simulink model "lesson_1"  (R2016a)
settings: Solver=VariableStepAuto  StartTime=0.0  StopTime=10.0  RelTol=1e-3
values from neighbouring files (symbols this model uses):
  D = 1e-3    (= 0.001)    [initialization_for_lesson1.m]    (also in initialization_for_lesson4.m; initialization_for_lesson5.m)
  f = 50    [initialization_for_lesson1.m]    (also in initialization_for_lesson2.m; initialization_for_lesson4.m; initialization_for_lesson5.m)
  Fs = Vs*sqrt(2/3)/(2*pi*f)    [initialization_for_lesson1.m]    (also in initialization_for_lesson2.m = ims*Lm; initialization_for_lesson4.m; initialization_for_lesson5.m)
  fsw = 4e3    (= 4000)    [initialization_for_lesson1.m]    (also in initialization_for_lesson4.m; initialization_for_lesson5.m)
  J = 127    [initialization_for_lesson1.m]    (also in initialization_for_lesson4.m; initialization_for_lesson5.m)
  ki_id = (wni^2)*Lr*sigma    (= 491.599501999)    [initialization_for_lesson1.m]    (also in initialization_for_lesson4.m; initialization_for_lesson5.m)
  ki_iq = ki_id    (= 491.599501999)    [initialization_for_lesson1.m]    (also in initialization_for_lesson4.m; initialization_for_lesson5.m)
  ki_n = ((wnn^2)*J)/p    (= 25400)    [initialization_for_lesson1.m]    (also in initialization_for_lesson4.m = 406400; initialization_for_lesson5.m = 406400)
  kp_id = (2*wni*sigma*Lr)-Rr    (= 0.5771)    [initialization_for_lesson1.m]    (also in initialization_for_lesson4.m; initialization_for_lesson5.m)
  kp_iq = kp_id    (= 0.5771)    [initialization_for_lesson1.m]    (also in initialization_for_lesson4.m; initialization_for_lesson5.m)
  kp_n = (2*wnn*J)/p    (= 2540)    [initialization_for_lesson1.m]    (also in initialization_for_lesson4.m = 10160; initialization_for_lesson5.m = 10160)
  Lm = 2.5e-3    (= 0.0025)    [initialization_for_lesson1.m]    (also in initialization_for_lesson2.m; initialization_for_lesson4.m; initialization_for_lesson5.m)
  Lr = Lm + Lsi    (= 0.002587)    [initialization_for_lesson1.m]    (also in initialization_for_lesson2.m; initialization_for_lesson4.m; initialization_for_lesson5.m)
  Ls = Lm + Lsi    (= 0.002587)    [initialization_for_lesson1.m]    (also in initialization_for_lesson2.m; initialization_for_lesson4.m; initialization_for_lesson5.m)
  Lsi = 0.087e-3    (= 8.7e-05)    [initialization_for_lesson1.m]    (also in initialization_for_lesson2.m; initialization_for_lesson4.m; initialization_for_lesson5.m)
  p = 2    [initialization_for_lesson1.m]    (also in initialization_for_lesson2.m; initialization_for_lesson4.m; initialization_for_lesson5.m)
  Ps = 2e6    (= 2000000)    [initialization_for_lesson1.m]    (also in initialization_for_lesson2.m; initialization_for_lesson4.m; initialization_for_lesson5.m)
  Rr = 2.9e-3    (= 0.0029)    [initialization_for_lesson1.m]    (also in initialization_for_lesson2.m; initialization_for_lesson4.m; initialization_for_lesson5.m)
  Rs = 2.6e-3    (= 0.0026)    [initialization_for_lesson1.m]    (also in initialization_for_lesson2.m; initialization_for_lesson4.m; initialization_for_lesson5.m)
  sigma = 1 - Lm^2/(Ls*Lr)    (= 0.0661284179513)    [initialization_for_lesson1.m]    (also in initialization_for_lesson2.m; initialization_for_lesson4.m; initialization_for_lesson5.m)
  Tem = 12732    [initialization_for_lesson1.m]    (also in initialization_for_lesson2.m = Temm(i); initialization_for_lesson4.m; initialization_for_lesson5.m)
  Ts = 1/fsw/50    (= 5e-06)    [initialization_for_lesson1.m]    (also in initialization_for_lesson4.m; initialization_for_lesson5.m)
  Vbus = Vr_stator*sqrt(2)    [initialization_for_lesson1.m]    (also in initialization_for_lesson2.m; initialization_for_lesson4.m; initialization_for_lesson5.m)
  Vs = 690    [initialization_for_lesson1.m]    (also in initialization_for_lesson2.m = 690*sqrt(2/3); initialization_for_lesson4.m; initialization_for_lesson5.m)
undefined symbols (not defined in the file or in its folder): DiscIntNeverNeededParam
libraries: powerlib x8, powerlib_meascontrol x1
settings Model: Creator=EBUKA  LastModifiedBy=EBUKA
settings GRTTargetCC: GeneratePreprocessorConditionals=Use local settings

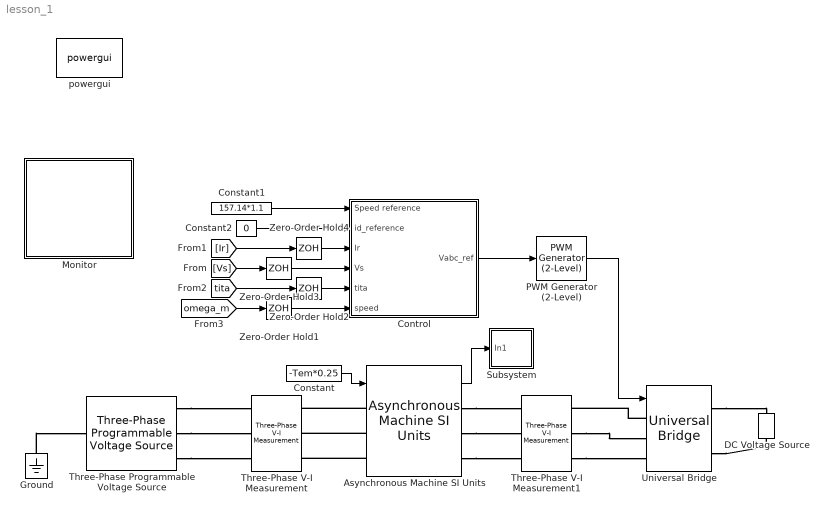
== system lesson_1 ==
  Asynchronous Machine SI Units : powerlib/Machines/Asynchronous Machine SI Units  RotorType=Wound  PresetModel=No  MechanicalLoad=Torque Tm  ShowDetailedParameters=on  ReferenceFrame=Rotor  Units=SI  MeasurementBus=off  NominalParameters=[Ps Vs f]  Stator=[Rs, Lsi]  Rotor=[Rr, Lsi]  Cage1=[0.4155 0.002066]  Cage2=[0.4168 0.0003495]  Lm=Lm  Mechanical=[J D 2]  PolePairs=2  InitialConditions=[1 0 0 0 0 0 0 0]  SimulateSaturation=off  Saturation=[14.03593122, 27.81365428, 53.79336849, 72.68890987, 97.98006896, 148.6815601, 215.7428561, 302.9841135, 428.7778367 ; 230, 322, 414, 460, 506, 552, 598, 644, 690]  LoadFlowParameters=1492000  TsPowergui=0  TsBlock=-1  IterativeModel=Trapezoidal non iterative  IterativeDiscreteModel=Trapezoidal non iterative  Pmec=1.492e+006
  Constant : Constant  Value=-Tem*0.25
  Constant1 : Constant  Value=157.14*1.1
  Constant2 : Constant  Value=0
  Control : Subsystem
  DC Voltage Source : powerlib/Electrical Sources/DC Voltage Source  Amplitude=Vbus  Measurements=None
  Ground : powerlib/Elements/Ground  LConnTagsString=a
  Monitor : Subsystem
  PWM Generator (2-Level) : powerlib_meascontrol/Pulse & Signal Generators/PWM Generator (2-Level)  ModulatorType=Three-phase bridge (6 pulses)  ModulatorMode=Unsynchronized  Fc=fsw  Pc=90  nF=27  MinMax="[ -1  1 ]"  SamplingTechnique=Symmetrical regular (single edge)  ModulatingSignals=off  m=0.8  Freq=60  Phase=0  Ts=0  ShowCarrierOutport=off
  Subsystem : Subsystem
  Three-Phase Programmable Voltage Source : powerlib/Electrical Sources/Three-Phase Programmable Voltage Source  PositiveSequence="[Vs  0 f]"  VariationEntity=None  VariationType=Table of time-amplitude pairs  VariationTypeAlt=Step  VariationStep=0.5  VariationRate=10  VariationMagnitude=0.3  VariationFrequency=2  VariationTiming=[1 2]  VariationPhaseA=off  Amplitudes=[1 0.8 1.2 1.0]  TimeValues=[0 0.1 0.15 0.2]  HarmonicGeneration=off  HarmonicA=[3 0.2 -25 0]  HarmonicB=[2 0.15 35 2]  Timing="[0.05  3]"  BusType=swing  Pref=0  Qref=0  Qmin=-inf  Qmax=inf
  Three-Phase V-I Measurement : powerlib/Measurements/Three-Phase V-I Measurement  VoltageMeasurement=phase-to-ground  SetLabelV=on  LabelV=Vs  Vpu=on  VpuLL=off  CurrentMeasurement=yes  SetLabelI=on  LabelI=Is  Ipu=off  Pbase=100e6  Vbase=500e3  OutputType=Complex  PhasorSimulation=off  PSBequivalent=0
  Three-Phase V-I Measurement1 : powerlib/Measurements/Three-Phase V-I Measurement  VoltageMeasurement=no  SetLabelV=off  LabelV=Vs  Vpu=off  VpuLL=off  CurrentMeasurement=yes  SetLabelI=on  LabelI=Ir  Ipu=off  Pbase=100e6  Vbase=500e3  OutputType=Complex  PhasorSimulation=off  PSBequivalent=0
  Universal Bridge : powerlib/Power Electronics/Universal Bridge  Arms=3  SnubberResistance=1e5  SnubberCapacitance=inf  Device=Ideal Switches  Ron=1e-3  Lon=0  ForwardVoltages="[  0  0  ]"  ForwardVoltage=0  GTOparameters=[ 10e-6 , 20e-6 ]  IGBTparameters=[ 1e-6 , 2e-6 ]  Measurements=None  Measurements_2=None  converterType=Rectifier
  Zero-Order Hold{1..4} (4 alike) : ZeroOrderHold  SampleTime=1/fsw
  powergui : powerlib/powergui  Priority=1  SimulationMode=Discrete  SolverType=Tustin/Backward Euler (TBE)  SampleTime=Ts  frequency=60  SPID=off  DisableSnubberDevices=off  DisableRonSwitches=off  DisableVfSwitches=off  SwTol=0  DisplayEquations=off  Interpol=off  ExternalGateDelay=off  methode=off  Ts=10  FunctionMessages=off  echomessages=off  HookPort=off  EnableUseOfTLC=off  x0status=blocks  frequencyindice=50  Pbase=100e6  ErrMax=1e-4  Iterations=50  UnitsV=kV  UnitsW=MW  buscounter=0  RestoreLinks=warning  ResistiveCurrentMeasurement=off  Frange=[0:2:500]  Ylog=off  Xlog=on  ShowGrid=off  save=off  variable=ZData  structure=0  ZoomFFT=off  StartTime=0.0  cycles=1  DisplayStyle=1  fundamental=60  FreqAxis=off  MaxFrequency=1000  frequencyindicesteady=1  RmsSteady=1  display=off
  wires:
  Constant/1 -> Asynchronous Machine SI Units/1
  PWM Generator (2-Level)/1 -> Universal Bridge/1
  Control/1(Vabc_ref) -> PWM Generator (2-Level)/1
  Constant1/1 -> Control/1(Speed reference)
  Constant2/1 -> Control/2(id_reference)
  [Vs] -> Zero-Order Hold3/1
  [Ir] -> Zero-Order Hold4/1
  Asynchronous Machine SI Units/1 -> Subsystem/1(In1)
  [tita] -> Zero-Order Hold2/1
  [omega_m] -> Zero-Order Hold1/1
  Zero-Order Hold2/1 -> Control/5(tita)
  Zero-Order Hold1/1 -> Control/6(speed)
  Zero-Order Hold3/1 -> Control/4(Vs)
  Zero-Order Hold4/1 -> Control/3(Ir)
  connections:
  Asynchronous Machine SI Units/LConn1 -- Three-Phase V-I Measurement/RConn1
  Asynchronous Machine SI Units/LConn2 -- Three-Phase V-I Measurement/RConn2
  Asynchronous Machine SI Units/LConn3 -- Three-Phase V-I Measurement/RConn3
  Three-Phase Programmable Voltage Source/RConn1 -- Three-Phase V-I Measurement/LConn1
  Three-Phase Programmable Voltage Source/RConn2 -- Three-Phase V-I Measurement/LConn2
  Three-Phase Programmable Voltage Source/RConn3 -- Three-Phase V-I Measurement/LConn3
  Ground/LConn1 -- Three-Phase Programmable Voltage Source/LConn1
  Universal Bridge/RConn2 -- DC Voltage Source/LConn1
  Universal Bridge/RConn1 -- DC Voltage Source/RConn1
  Asynchronous Machine SI Units/RConn1 -- Three-Phase V-I Measurement1/RConn1
  Asynchronous Machine SI Units/RConn2 -- Three-Phase V-I Measurement1/RConn2
  Asynchronous Machine SI Units/RConn3 -- Three-Phase V-I Measurement1/RConn3
  Universal Bridge/LConn1 -- Three-Phase V-I Measurement1/LConn1
  Three-Phase V-I Measurement1/LConn2 -- Universal Bridge/LConn2
  Three-Phase V-I Measurement1/LConn3 -- Universal Bridge/LConn3

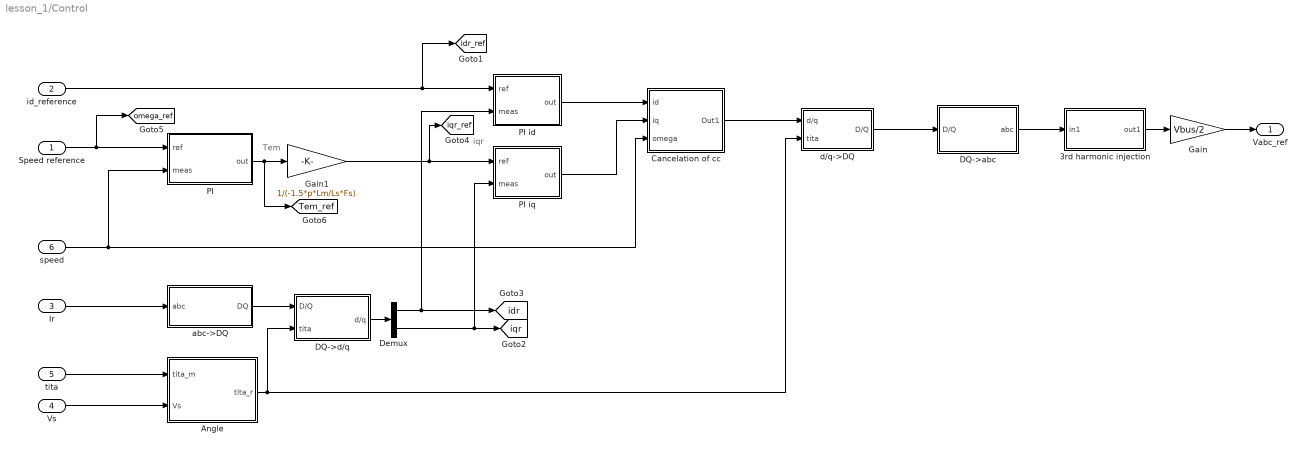
== system lesson_1/Control ==
  note: iqr
  note: Tem
  Speed reference : Inport
  id_reference : Inport  Port=2
  Ir : Inport  Port=3
  Vs : Inport  Port=4
  tita : Inport  Port=5
  speed : Inport  Port=6
  3rd harmonic injection : Subsystem
  Angle : Subsystem
  Cancelation of cc : Subsystem
  DQ->abc : Subsystem
  DQ->d/q : Subsystem
  Demux : Demux  Outputs=2
  Gain : Gain  Gain=Vbus/2
  Gain1 : Gain  Gain=1/(-1.5*p*Lm/Ls*Fs)
  PI : Subsystem
  PI id : Subsystem
  PI iq : Subsystem
  abc->DQ : Subsystem
  d/q->DQ : Subsystem
  Vabc_ref : Outport
  tag scope: Tem_ref=global, idr=global, idr_ref=global, iqr=global, iqr_ref=global, omega_ref=global
  wires:
  DQ->abc/1(abc) -> 3rd harmonic injection/1(in1)
  Gain/1 -> Vabc_ref/1
  d/q->DQ/1(D/Q) -> DQ->abc/1(D/Q)
  Ir/1 -> abc->DQ/1(abc)
  abc->DQ/1(DQ) -> DQ->d/q/1(D/Q)
  3rd harmonic injection/1(out1) -> Gain/1
  tita/1 -> Angle/1(tita_m)
  Vs/1 -> Angle/2(Vs)
  PI id/1(out) -> Cancelation of cc/1(id)
  PI iq/1(out) -> Cancelation of cc/2(iq)
  speed/1 -> PI/2(meas), Cancelation of cc/3(omega)
  Cancelation of cc/1(Out1) -> d/q->DQ/1(d/q)
  DQ->d/q/1(d/q) -> Demux/1
  Demux/1 -> [idr], PI id/2(meas)
  Demux/2 -> [iqr], PI iq/2(meas)
  Speed reference/1 -> [omega_ref], PI/1(ref)
  Angle/1(tita_r) -> d/q->DQ/2(tita), DQ->d/q/2(tita)
  PI/1(out) -> [Tem_ref], Gain1/1
  Gain1/1 -> [iqr_ref], PI iq/1(ref)
  id_reference/1 -> [idr_ref], PI id/1(ref)

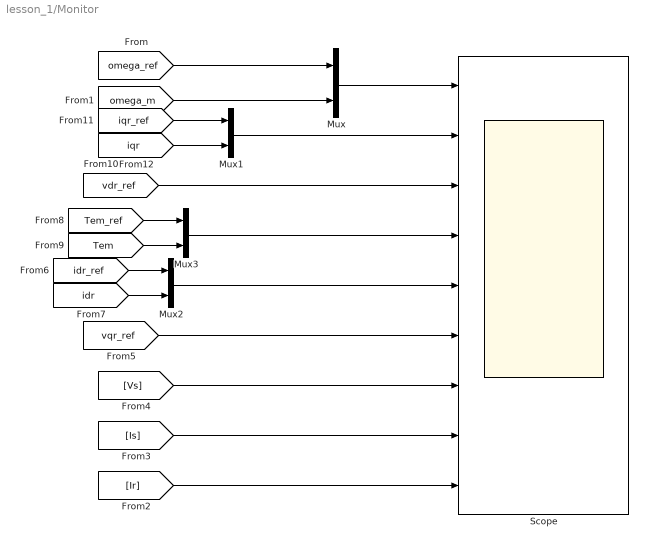
== system lesson_1/Monitor ==
  Mux{,1..3} (4 alike) : Mux  Inputs=2
  Scope : Scope  NumInputPorts=9
  wires:
  [omega_ref] -> Mux/1
  [omega_m] -> Mux/2
  [Ir] -> Scope/9
  [Is] -> Scope/8
  [Vs] -> Scope/7
  [idr_ref] -> Mux2/1
  [idr] -> Mux2/2
  Mux3/1 -> Scope/4
  [Tem_ref] -> Mux3/1
  [Tem] -> Mux3/2
  [vdr_ref] -> Scope/3
  [iqr_ref] -> Mux1/1
  [iqr] -> Mux1/2
  Mux1/1 -> Scope/2
  Mux2/1 -> Scope/5
  [vqr_ref] -> Scope/6
  Mux/1 -> Scope/1

== system lesson_1/Subsystem ==
  In1 : Inport
  Bus Selector : BusSelector  OutputSignals=Mechanical.Rotor angle thetam (rad),Mechanical.Rotor speed (wm),Mechanical.Electromagnetic torque Te (N*m)
  tag scope: Tem=global, omega_m=global, tita=global
  wires:
  In1/1 -> Bus Selector/1
  Bus Selector/2 -> [omega_m]  "<Rotor speed (wm)>"
  Bus Selector/1 -> [tita]  "<Rotor angle thetam (rad)>"
  Bus Selector/3 -> [Tem]  "<Electromagnetic torque Te (N*m)>"

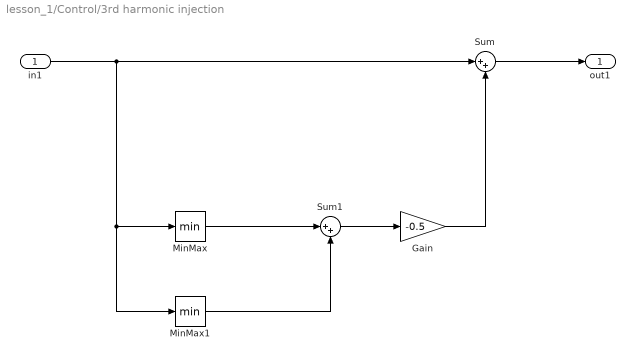
== system lesson_1/Control/3rd harmonic injection ==
  in1 : Inport
  Gain : Gain  Gain=-0.5
  MinMax : MinMax
  MinMax1 : MinMax
  Sum : Sum  Inputs=|++
  Sum1 : Sum  Inputs=|++
  out1 : Outport
  wires:
  Sum/1 -> out1/1
  in1/1 -> MinMax1/1, MinMax/1, Sum/1
  Gain/1 -> Sum/2
  Sum1/1 -> Gain/1
  MinMax/1 -> Sum1/1
  MinMax1/1 -> Sum1/2

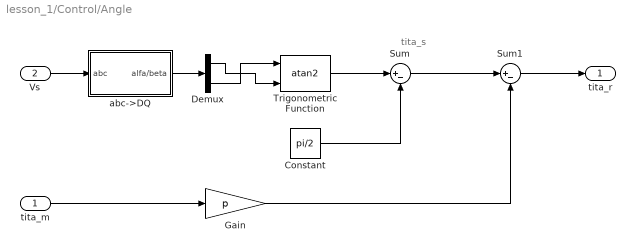
== system lesson_1/Control/Angle ==
  note: tita_s
  tita_m : Inport
  Vs : Inport  Port=2
  Constant : Constant  Value=pi/2
  Demux : Demux  Outputs=2
  Gain : Gain  Gain=p
  Sum : Sum  Inputs=|+-
  Sum1 : Sum  Inputs=|+-
  Trigonometric Function : Trigonometry  Operator=atan2
  abc->DQ : Subsystem
  tita_r : Outport
  wires:
  Vs/1 -> abc->DQ/1(abc)
  abc->DQ/1(alfa/beta) -> Demux/1
  Demux/2 -> Trigonometric Function/1
  Demux/1 -> Trigonometric Function/2
  Trigonometric Function/1 -> Sum/1
  Constant/1 -> Sum/2
  Sum/1 -> Sum1/1
  tita_m/1 -> Gain/1
  Sum1/1 -> tita_r/1
  Gain/1 -> Sum1/2

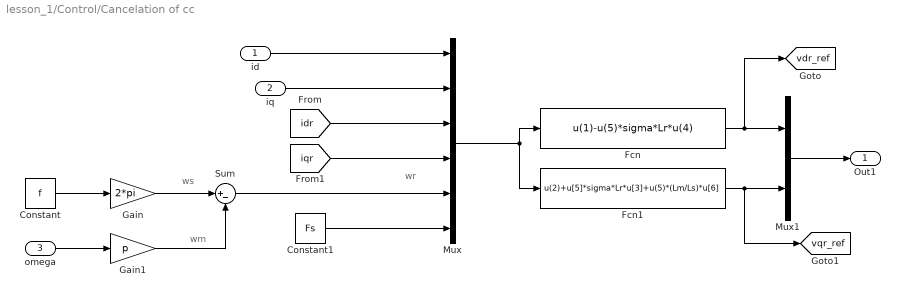
== system lesson_1/Control/Cancelation of cc ==
  note: wm
  note: ws
  note: wr
  id : Inport
  iq : Inport  Port=2
  omega : Inport  Port=3
  Constant : Constant  Value=f
  Constant1 : Constant  Value=Fs
  Fcn : Fcn  Expr=u(1)-u(5)*sigma*Lr*u(4)
  Fcn1 : Fcn  Expr=u(2)+u[5]*sigma*Lr*u[3]+u(5)*(Lm/Ls)*u[6]
  Gain : Gain  Gain=2*pi
  Gain1 : Gain  Gain=p
  Mux : Mux  Inputs=6
  Mux1 : Mux  Inputs=2
  Sum : Sum  Inputs=|+-
  Out1 : Outport
  tag scope: vdr_ref=global, vqr_ref=global
  wires:
  Mux/1 -> Fcn/1, Fcn1/1
  Fcn/1 -> [vdr_ref], Mux1/1
  Fcn1/1 -> [vqr_ref], Mux1/2
  Mux1/1 -> Out1/1
  id/1 -> Mux/1
  iq/1 -> Mux/2
  [idr] -> Mux/3
  [iqr] -> Mux/4
  Constant/1 -> Gain/1
  Gain/1 -> Sum/1
  Sum/1 -> Mux/5
  omega/1 -> Gain1/1
  Gain1/1 -> Sum/2
  Constant1/1 -> Mux/6

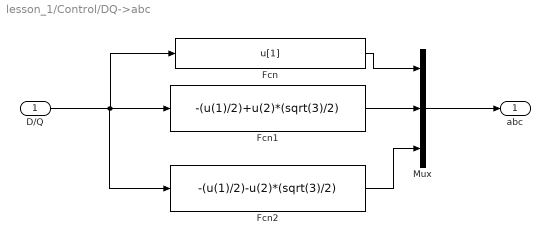
== system lesson_1/Control/DQ->abc ==
  D/Q : Inport
  Fcn : Fcn  Expr=u[1]
  Fcn1 : Fcn  Expr=-(u(1)/2)+u(2)*(sqrt(3)/2)
  Fcn2 : Fcn  Expr=-(u(1)/2)-u(2)*(sqrt(3)/2)
  Mux : Mux  Inputs=3
  abc : Outport
  wires:
  Mux/1 -> abc/1
  Fcn/1 -> Mux/1
  Fcn1/1 -> Mux/2
  Fcn2/1 -> Mux/3
  D/Q/1 -> Fcn2/1, Fcn1/1, Fcn/1

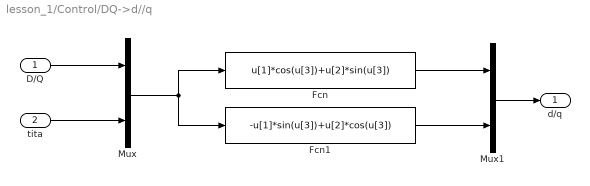
== system lesson_1/Control/DQ->d//q ==
  D/Q : Inport
  tita : Inport  Port=2
  Fcn : Fcn  Expr=u[1]*cos(u[3])+u[2]*sin(u[3])
  Fcn1 : Fcn  Expr=-u[1]*sin(u[3])+u[2]*cos(u[3])
  Mux : Mux  Inputs=2
  Mux1 : Mux  Inputs=2
  d/q : Outport
  wires:
  D/Q/1 -> Mux/1
  tita/1 -> Mux/2
  Mux1/1 -> d/q/1
  Fcn/1 -> Mux1/1
  Fcn1/1 -> Mux1/2
  Mux/1 -> Fcn1/1, Fcn/1

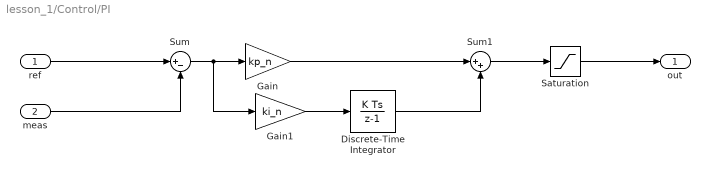
== system lesson_1/Control/PI ==
  ref : Inport
  meas : Inport  Port=2
  Discrete-Time Integrator : DiscreteIntegrator  InitialConditionSetting=State (most efficient)  SampleTime=1/fsw  LimitOutput=on  UpperSaturationLimit=Tem  LowerSaturationLimit=-Tem  ICPrevOutput=DiscIntNeverNeededParam  ICPrevScaledInput=DiscIntNeverNeededParam
  Gain : Gain  Gain=kp_n
  Gain1 : Gain  Gain=ki_n
  Saturation : Saturate  UpperLimit=Tem  LowerLimit=-Tem
  Sum : Sum  Inputs=|+-
  Sum1 : Sum  Inputs=|++
  out : Outport
  wires:
  ref/1 -> Sum/1
  meas/1 -> Sum/2
  Sum/1 -> Gain1/1, Gain/1
  Sum1/1 -> Saturation/1
  Gain/1 -> Sum1/1
  Saturation/1 -> out/1
  Gain1/1 -> Discrete-Time Integrator/1
  Discrete-Time Integrator/1 -> Sum1/2

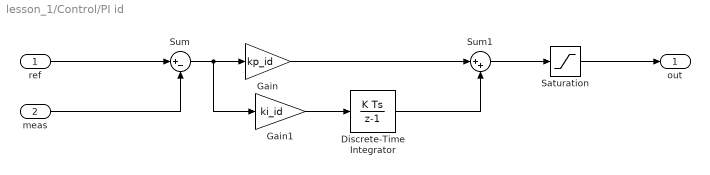
== system lesson_1/Control/PI id ==
  ref : Inport
  meas : Inport  Port=2
  Discrete-Time Integrator : DiscreteIntegrator  InitialConditionSetting=State (most efficient)  SampleTime=1/fsw  LimitOutput=on  UpperSaturationLimit=Vbus/sqrt(3)  LowerSaturationLimit=-Vbus/sqrt(3)  ICPrevOutput=DiscIntNeverNeededParam  ICPrevScaledInput=DiscIntNeverNeededParam
  Gain : Gain  Gain=kp_id
  Gain1 : Gain  Gain=ki_id
  Saturation : Saturate  UpperLimit=Vbus/sqrt(3)  LowerLimit=-Vbus/sqrt(3)
  Sum : Sum  Inputs=|+-
  Sum1 : Sum  Inputs=|++
  out : Outport
  wires:
  ref/1 -> Sum/1
  meas/1 -> Sum/2
  Sum/1 -> Gain1/1, Gain/1
  Sum1/1 -> Saturation/1
  Gain/1 -> Sum1/1
  Saturation/1 -> out/1
  Gain1/1 -> Discrete-Time Integrator/1
  Discrete-Time Integrator/1 -> Sum1/2

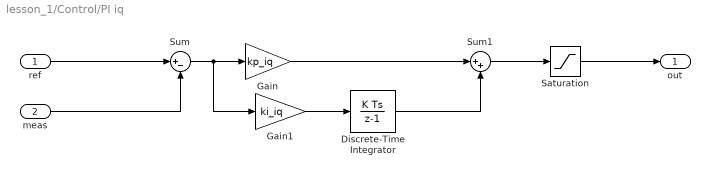
== system lesson_1/Control/PI iq ==
  ref : Inport
  meas : Inport  Port=2
  Discrete-Time Integrator : DiscreteIntegrator  InitialConditionSetting=State (most efficient)  SampleTime=1/fsw  LimitOutput=on  UpperSaturationLimit=Vbus/sqrt(3)  LowerSaturationLimit=-Vbus/sqrt(3)  ICPrevOutput=DiscIntNeverNeededParam  ICPrevScaledInput=DiscIntNeverNeededParam
  Gain : Gain  Gain=kp_iq
  Gain1 : Gain  Gain=ki_iq
  Saturation : Saturate  UpperLimit=Vbus/sqrt(3)  LowerLimit=-Vbus/sqrt(3)
  Sum : Sum  Inputs=|+-
  Sum1 : Sum  Inputs=|++
  out : Outport
  wires:
  ref/1 -> Sum/1
  meas/1 -> Sum/2
  Sum/1 -> Gain1/1, Gain/1
  Sum1/1 -> Saturation/1
  Gain/1 -> Sum1/1
  Saturation/1 -> out/1
  Gain1/1 -> Discrete-Time Integrator/1
  Discrete-Time Integrator/1 -> Sum1/2

== system lesson_1/Control/abc->DQ ==
  abc : Inport
  Fcn : Fcn  Expr=2/3*(u[1]-u(2)/2-u(3)/2)
  Fcn1 : Fcn  Expr=2/3*(u(2)*(sqrt(3)/2)-u(3)*(sqrt(3)/2))
  Mux : Mux  Inputs=2
  DQ : Outport
  wires:
  Fcn/1 -> Mux/1
  Mux/1 -> DQ/1
  Fcn1/1 -> Mux/2
  abc/1 -> Fcn1/1, Fcn/1

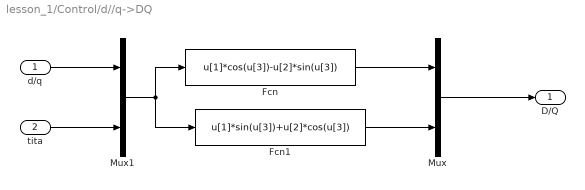
== system lesson_1/Control/d//q->DQ ==
  d/q : Inport
  tita : Inport  Port=2
  Fcn : Fcn  Expr=u[1]*cos(u[3])-u[2]*sin(u[3])
  Fcn1 : Fcn  Expr=u[1]*sin(u[3])+u[2]*cos(u[3])
  Mux : Mux  Inputs=2
  Mux1 : Mux  Inputs=2
  D/Q : Outport
  wires:
  d/q/1 -> Mux1/1
  tita/1 -> Mux1/2
  Mux/1 -> D/Q/1
  Fcn/1 -> Mux/1
  Fcn1/1 -> Mux/2
  Mux1/1 -> Fcn1/1, Fcn/1

== system lesson_1/Control/Angle/abc->DQ ==
  abc : Inport
  Fcn : Fcn  Expr=2/3*(u[1]-u(2)/2-u(3)/2)
  Fcn1 : Fcn  Expr=2/3*(u(2)*(sqrt(3)/2)-u(3)*(sqrt(3)/2))
  Mux : Mux  Inputs=2
  alfa/beta : Outport
  wires:
  Fcn/1 -> Mux/1
  Mux/1 -> alfa/beta/1
  Fcn1/1 -> Mux/2
  abc/1 -> Fcn1/1, Fcn/1
